simulink model "anfismicrogrid"  (R2017a)
settings: Solver=ode45  StartTime=0.0  StopTime=1  RelTol=1e-3  EnableMultiTasking=on
undefined symbols (not defined in the file or in its folder): idq, idq1, PV1
libraries: powerlib x57, powerlib_meascontrol x5, fuzblock x4, powerlib_extras x3, simulink x1, re_lib x1
(part 1 of 2)
settings Model: Creator=Indhu  LastModifiedBy=venka
settings DataIOCC: LimitDataPoints=on  SaveFormat=Array
settings OptimizationCC: LifeSpan=inf
settings DebuggingCC: SolverPrmCheckMsg=warning  SFUnexpectedBacktrackingDiag=warning  SFNoUnconditionalDefaultTransitionDiag=warning  SFExecutionAtInitializationDiag=none
settings HardwareCC: ProdBitPerPointer=32  ProdBitPerSizeT=32  ProdBitPerPtrDiffT=32  ProdLargestAtomicFloat=None  ProdIntDivRoundTo=Undefined  ProdEndianess=Unspecified  ProdWordSize=32  ProdHWDeviceType=32-bit Generic
settings ModelReferenceCC: PropagateSignalLabelsOutOfModel=off
settings GRTTargetCC: TargetLangStandard=C89/C90 (ANSI)  GeneratePreprocessorConditionals=Disable all
settings ConfigComp: CovMetricSettings=dw  CovHtmlReporting=on  CovSaveCumulativeToWorkspaceVar=on  CovSaveSingleToWorkspaceVar=on  CovExternalEMLEnable=off  CovSFcnEnable=off

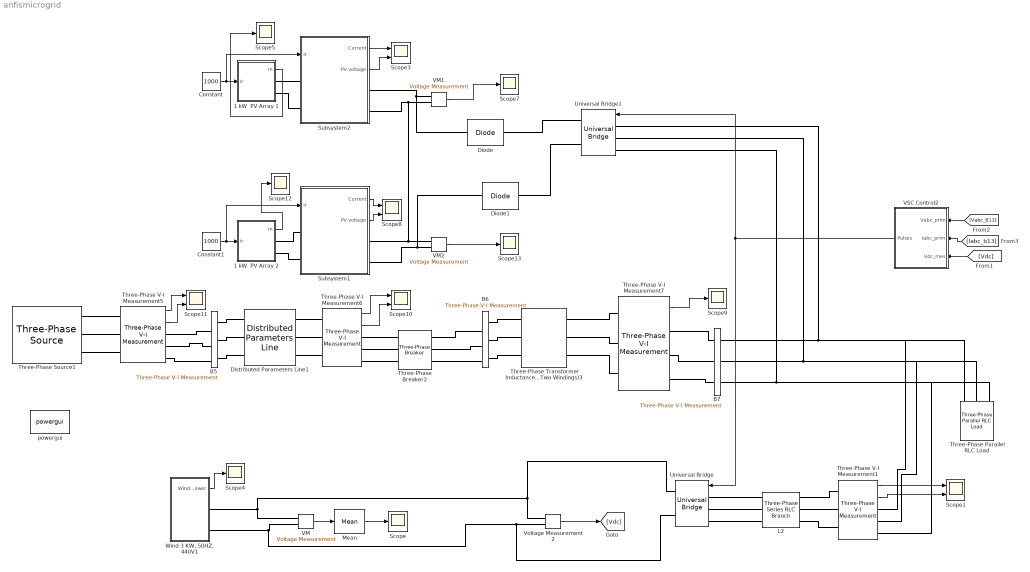
== system anfismicrogrid ==
  1 kW  PV Array 1 : Subsystem  mask(PV array){ModuleType=Suntech STP270S-24_Vb, Ncell=72, Nser=2, Npar=50, ModuleParameters=[ 44.4999  8.19978  35  7.70979 ], ModelParameters=[ 0.32025  2562.3  8.8992e-07  8.2979  1.5 ], Ts=10, PlotVI_module=off, PlotVI_array=off}
      mask prompts: ModuleType "Module type:"; Ncell "Number of cells per module"; Nser "Number of series-connected  modules per string"; Npar "Number of parallel strings"; ModuleParameters "Module specifications under STC  [  Voc, Isc, Vmp, Imp ]"; ModelParameters "Model parameters for 1 module [ Rs, Rp, Isat, Iph, Qd ]"; Ts "Sample time"; PlotVI_module "Display  I-V and  P-V characteritics of one module"; PlotVI_array "Display  I-V and  P-V characteritics of array"
      mask help:
      | Model a PV array
      |
      | PV array consists of Npar strings of modules connected in parallel, each string consisting of Nser modules connected in series.
      |
      | The four PV model parameters (photo-generated current Iph, diode saturation current Isat, parallel resistance Rp and  series resistance Rs) are adjuted to fit the following four module characteristics measured under standard test conditions (STC : irradiance 1000 W/m^2, cell temperature=25 deg. C) and assuming a given "diode quality factor" (Qd) for the semiconductor:
      |   Voc = open circuit voltage
      |   Isc = short-circuit current
      |   Vmp,Imp = voltage and current at maximum power point
      |
      | Select a 'Module type' and then press Apply to see module parameters.
      | Note: Module characteristics are extracted from NREL System Advisor Model.
      mask init:
      | BlockName=gcb;
      | 
      | % SolarModuleSpec_Definition_v2.m
      | %================================
      | %
      | Type=1;
      | SolarModuleSpec(Type).Desc= 'Kyocera KD135GX-LP';
      | SolarModuleSpec(Type).nCells= 36;              % Number of cells in series
      | SolarModuleSpec(Type).Pmp= 135.044;            % Maximum power (W)
      | SolarModuleSpec(Type).Vmp= 17.7;               % Maximum power voltage (V) 
      | SolarModuleSpec(Type).Imp= 7.62959;            % Maximum power current (A)
      | SolarModuleSpec(Type).Voc= 22.0999;            % Open circuit voltage (V)
      | SolarModuleSpec(Type).Isc= 8.36955;            % Short circuit current (A)
      | SolarModuleSpec(Type).TempC_Pmp= -6.445e-001;  % Maximum power temp. coefficient (W/deg.C)
      | SolarModuleSpec(Type).TempC_Vmp= -8.200e-002;  % Maximum power voltage temp. coefficient (V/deg.C)
      | SolarModuleSpec(Type).TempC_Imp= -1.068e-003;  % Maximum power current temp. coefficient (A/deg.C
      | SolarModuleSpec(Type).TempC_Voc= -8.000e-002;  % Open circuit voltage temp. coefficient (V/deg.C)
      | SolarModuleSpec(Type).TempC_Isc= 5.022e-003;   % Short circuit current temp. coefficient (A/deg.C)
      | SolarModuleSpec(Type).Rs= 0.10593;             % Series resistance of PV model (ohms)
      | SolarModuleSpec(Type).Rp= 142.84;              % Parallel resistance of PV model (ohms)
      | SolarModuleSpec(Type).Isat= 9.845e-07;         % Diode saturation current of PV model (A)
      | SolarModuleSpec(Type).Iph=  8.3758;            % Light-generated photo-current  of PV model (A)
      | SolarModuleSpec(Type).Qd= 1.5;                 % Diode quality factor of PV model
      | %-------------------------------------------------------------------------
      | %
      | Type=2;
      | SolarModuleSpec(Type).Desc= 'Kyocera KD205GX-LP';
      | SolarModuleSpec(Type).nCells= 54;              % Number of cells in series
      | SolarModuleSpec(Type).Pmp= 205.075;            % Maximum power (W)
      | SolarModuleSpec(Type).Vmp= 26.6;               % Maximum power voltage (V) 
      | SolarModuleSpec(Type).Imp= 7.70959;            % Maximum power current (A)
      | SolarModuleSpec(Type).Voc= 33.1999;            % Open circuit voltage (V)
      | SolarModuleSpec(Type).Isc= 8.35955;            % Short circuit current (A)
      | SolarModuleSpec(Type).TempC_Pmp= -9.770e-001;  % Maximum power temp. coefficient (W/deg.C)
      | SolarModuleSpec(Type).TempC_Vmp= -1.230e-001;  % Maximum power voltage temp. coefficient (V/deg.C)
      | SolarModuleSpec(Type).TempC_Imp= -1.079e-003;  % Maximum power current temp. coefficient (A/deg.C
      | SolarModuleSpec(Type).TempC_Voc= -1.200e-001;  % Open circuit voltage temp. coefficient (V/deg.C)
      | SolarModuleSpec(Type).TempC_Isc= 5.016e-003;   % Short circuit current temp. coefficient (A/deg.C)
      | SolarModuleSpec(Type).Rs= 0.15945;             % Series resistance of PV model (ohms)
      | SolarModuleSpec(Type).Rp= 1010.6;              % Parallel resistance of PV model (ohms)
      | SolarModuleSpec(Type).Isat=  9.7399e-07;       % Diode saturation current of PV model (A)
      | SolarModuleSpec(Type).Iph= 8.3642;             % Light-generated photo-current  of PV model (A)
      | SolarModuleSpec(Type).Qd= 1.5;                 % Diode quality factor of PV model
      | %-------------------------------------------------------------------------
      | %
      | Type=3;
      | SolarModuleSpec(Type).Desc= 'Mitsubishi PV-UD190MF5';
      | SolarModuleSpec(Type).nCells= 50;              % Number of cells in series
      | SolarModuleSpec(Type).Pmp= 190.503;            % Maximum power (W)
      | SolarModuleSpec(Type).Vmp= 24.6999;            % Maximum power voltage (V) 
      | SolarModuleSpec(Type).Imp= 7.71272;            % Maximum power current (A)
      | SolarModuleSpec(Type).Voc= 30.8006;            % Open circuit voltage (V)
      | SolarModuleSpec(Type).Isc= 8.23289;            % Short circuit current (A)
      | SolarModuleSpec(Type).TempC_Pmp= -8.597e-001;  % Maximum power temp. coefficient (W/deg.C)
      | SolarModuleSpec(Type).TempC_Vmp= -1.090e-001;  % Maximum power voltage temp. coefficient (V/deg.C)
      | SolarModuleSpec(Type).TempC_Imp= -7.713e-004;  % Maximum power current temp. coefficient (A/deg.C
      | SolarModuleSpec(Type).TempC_Voc= -1.050e-001;  % Open circuit voltage temp. coefficient (V/deg.C)
      | SolarModuleSpec(Type).TempC_Isc= 4.446e-003;   % Short circuit current temp. coefficient (A/deg.C)
      | SolarModuleSpec(Type).Rs= 0.20758;             % Series resistance of PV model (ohms)
      | SolarModuleSpec(Type).Rp= 975.6;               % Parallel resistance of PV model (ohms)
      | SolarModuleSpec(Type).Isat= 7.9676e-08;        % Diode saturation current of PV model (A)
      | SolarModuleSpec(Type).Iph= 8.2649;             % Light-generated photo-current  of PV model (A)
      | SolarModuleSpec(Type).Qd= 1.3;                 % Diode quality factor of PV model
      | %-------------------------------------------------------------------------
      | %
      | Type=4;
      | SolarModuleSpec(Type).Desc= 'Sanyo HIP-225HDE1';
      | SolarModuleSpec(Type).nCells= 60;              % Number of cells in series
      | SolarModuleSpec(Type).Pmp= 224.899;            % Maximum power (W)
      | SolarModuleSpec(Type).Vmp= 33.9;               % Maximum power voltage (V) 
      | SolarModuleSpec(Type).Imp= 6.63419;            % Maximum power current (A)
      | SolarModuleSpec(Type).Voc= 41.7984;            % Open circuit voltage (V)
      | SolarModuleSpec(Type).Isc= 7.13383;            % Short circuit current (A)
      | SolarModuleSpec(Type).TempC_Pmp= -6.925e-001;  % Maximum power temp. coefficient (W/deg.C)
      | SolarModuleSpec(Type).TempC_Vmp= -1.010e-001;  % Maximum power voltage temp. coefficient (V/deg.C)
      | SolarModuleSpec(Type).TempC_Imp= -6.634e-004;  % Maximum power current temp. coefficient (A/deg.C
      | SolarModuleSpec(Type).TempC_Voc= -1.050e-001;  % Open circuit voltage temp. coefficient (V/deg.C)
      | SolarModuleSpec(Type).TempC_Isc= 2.140e-003;   % Short circuit current temp. coefficient (A/deg.C)
      | SolarModuleSpec(Type).Rs=  0.20439;            % Series resistance of PV model (ohms)
      | SolarModuleSpec(Type).Rp= 1830.7;              % Parallel resistance of PV model (ohms)
      | SolarModuleSpec(Type).Isat=  3.0815e-07;       % Diode saturation current of PV model (A)
      | SolarModuleSpec(Type).Iph=  7.145;             % Light-generated photo-current  of PV model (A)
      | SolarModuleSpec(Type).Qd= 1.6;                 % Diode quality factor of PV model
      | %-------------------------------------------------------------------------
      | %
      | 
      | Type=5;
      | % NREL : 2007(E)
      | SolarModuleSpec(Type).Desc= 'SunPower SPR-305-WHT';
      | SolarModuleSpec(Type).nCells= 96;              % Number of cells in series
      | SolarModuleSpec(Type).Pmp= 305.2;              % Maximum power (W)
      | SolarModuleSpec(Type).Vmp= 54.70;              % Maximum power voltage (V) 
      | SolarModuleSpec(Type).Imp= 5.58;               % Maximum power current (A)
      | SolarModuleSpec(Type).Voc= 64.20;              % Open circuit voltage (V)
      | SolarModuleSpec(Type).Isc= 5.96;               % Short circuit current (A)
      | SolarModuleSpec(Type).TempC_Pmp= -1.154e+000;  % Maximum power temp. coefficient (W/deg.C)
      | SolarModuleSpec(Type).TempC_Vmp= -1.860e-001;  % Maximum power voltage temp. coefficient (V/deg.C)
      | SolarModuleSpec(Type).TempC_Imp= -2.120e-003;  % Maximum power current temp. coefficient (A/deg.C
      | SolarModuleSpec(Type).TempC_Voc= -1.770e-001;  % Open circuit voltage temp. coefficient (V/deg.C)
      | SolarModuleSpec(Type).TempC_Isc= 3.516e-003;   % Short circuit current temp. coefficient (A/deg.C)
      | SolarModuleSpec(Type).Rs= 0.037998;            % Series resistance of PV model (ohms)
      | SolarModuleSpec(Type).Rp= 993.51;              % Parallel resistance of PV model (ohms)
      | SolarModuleSpec(Type).Isat= 1.1753e-08;        % Diode saturation current of PV model (A)
      | SolarModuleSpec(Type).Iph= 5.9602;             % Light-generated photo-current  of PV model (A)
      | SolarModuleSpec(Type).Qd= 1.3;                 % Diode quality factor of PV model
      | %-------------------------------------------------------------------------
      | %
      | Type=6;
      | SolarModuleSpec(Type).Desc= 'Suntech STP270S-24_Vb';
      | SolarModuleSpec(Type).nCells= 72;              % Number of cells in series
      | SolarModuleSpec(Type).Pmp= 269.843;            % Maximum power (W)
      | SolarModuleSpec(Type).Vmp= 35;                 % Maximum power voltage (V) 
      | SolarModuleSpec(Type).Imp= 7.70979;            % Maximum power current (A)
      | SolarModuleSpec(Type).Voc= 44.4999;            % Open circuit voltage (V)
      | SolarModuleSpec(Type).Isc= 8.19978;            % Short circuit current (A)
      | SolarModuleSpec(Type).TempC_Pmp= -1.204e+000;  % Maximum power temp. coefficient (W/deg.C)
      | SolarModuleSpec(Type).TempC_Vmp= -1.567e-001;  % Maximum power voltage temp. coefficient (V/deg.C)
      | SolarModuleSpec(Type).TempC_Imp= 1.234e-004;   % Maximum power current temp. coefficient (A/deg.C
      | SolarModuleSpec(Type).TempC_Voc= -1.504e-001;  % Open circuit voltage temp. coefficient (V/deg.C)
      | SolarModuleSpec(Type).TempC_Isc= 4.969e-003;   % Short circuit current temp. coefficient (A/deg.C)
      | SolarModuleSpec(Type).Rs= 0.32025;             % Series resistance of PV model (ohms)
      | SolarModuleSpec(Type).Rp= 2562.3;              % Parallel resistance of PV model (ohms)
      | SolarModuleSpec(Type).Isat= 8.8992e-07;        % Diode saturation current of PV model (A)
      | SolarModuleSpec(Type).Iph= 8.2979;             % Light-generated photo-current  of PV model (A)
      | SolarModuleSpec(Type).Qd= 1.5;                 % Diode quality factor of PV model
      | % 
      | %-------------------------------------------------------------------------
      | %
      | Type=7;
      | SolarModuleSpec(Type).Desc= 'Canadian Solar CS5P-220M';
      | SolarModuleSpec(Type).nCells= 96;              % Number of cells in series
      | SolarModuleSpec(Type).Pmp= 219.72;             % Maximum power (W)
      | SolarModuleSpec(Type).Vmp= 48.3159;            % Maximum power voltage (V) 
      | SolarModuleSpec(Type).Imp= 4.54758;            % Maximum power current (A)
      | SolarModuleSpec(Type).Voc= 59.2618;            % Open circuit voltage (V)
      | SolarModuleSpec(Type).Isc= 5.09261;            % Short circuit current (A)
      | SolarModuleSpec(Type).TempC_Pmp= -1.031e+000;  % Maximum power temp. coefficient (W/deg.C)
      | SolarModuleSpec(Type).TempC_Vmp= -2.355e-001;  % Maximum power voltage temp. coefficient (V/deg.C)
      | SolarModuleSpec(Type).TempC_Imp= 8.231e-004;   % Maximum power current temp. coefficient (A/deg.C
      | SolarModuleSpec(Type).TempC_Voc= -2.170e-001;  % Open circuit voltage temp. coefficient (V/deg.C)
      | SolarModuleSpec(Type).TempC_Isc= 2.022e-003;   % Short circuit current temp. coefficient (A/deg.C)
      | SolarModuleSpec(Type).Rs= 0.24807;             % Series resistance of PV model (ohms)
      | SolarModuleSpec(Type).Rp= 235.76;              % Parallel resistance of PV model (ohms)
      | SolarModuleSpec(Type).Isat= 5.3103e-07;        % Diode saturation current of PV model (A)
      | SolarModuleSpec(Type).Iph= 5.098;              % Light-generated photo-current  of PV model (A)
      | SolarModuleSpec(Type).Qd= 1.5;                 % Diode quality factor of PV model
      | %-------------------------------------------------------------------------
      | %
      | Type=8;
      | SolarModuleSpec(Type).Desc= 'BP Solar SX3190';
      | SolarModuleSpec(Type).nCells= 50;              % Number of cells in series
      | SolarModuleSpec(Type).Pmp= 190.258;            % Maximum power (W)
      | SolarModuleSpec(Type).Vmp= 24.3003;            % Maximum power voltage (V) 
      | SolarModuleSpec(Type).Imp= 7.82945;            % Maximum power current (A)
      | SolarModuleSpec(Type).Voc= 30.6021;            % Open circuit voltage (V)
      | SolarModuleSpec(Type).Isc= 8.51029;            % Short circuit current (A)
      | SolarModuleSpec(Type).TempC_Pmp= -9.306e-001;  % Maximum power temp. coefficient (W/deg.C)
      | SolarModuleSpec(Type).TempC_Vmp= -1.140e-001;  % Maximum power voltage temp. coefficient (V/deg.C)
      | SolarModuleSpec(Type).TempC_Imp= -1.566e-003;  % Maximum power current temp. coefficient (A/deg.C
      | SolarModuleSpec(Type).TempC_Voc= -1.110e-001;  % Open circuit voltage temp. coefficient (V/deg.C)
      | SolarModuleSpec(Type).TempC_Isc= 5.532e-003;   % Short circuit current temp. coefficient (A/deg.C)
      | SolarModuleSpec(Type).Rs= 0.17514;             % Series resistance of PV model (ohms)
      | SolarModuleSpec(Type).Rp= 755.51;              % Parallel resistance of PV model (ohms)
      | SolarModuleSpec(Type).Isat= 1.0647e-06;       % Diode saturation current of PV model (A)
      | SolarModuleSpec(Type).Iph= 8.5158;             % Light-generated photo-current  of PV model (A)
      | SolarModuleSpec(Type).Qd= 1.5;                 % Diode quality factor of PV model
      | %-------------------------------------------------------------------------
      | %
      | Type=9;
      | SolarModuleSpec(Type).Desc= 'First Solar FS-272';
      | SolarModuleSpec(Type).nCells= 116;             % Number of cells in series
      | SolarModuleSpec(Type).Pmp= 71.326;             % Maximum power (W)
      | SolarModuleSpec(Type).Vmp= 70.558;             % Maximum power voltage (V) 
      | SolarModuleSpec(Type).Imp= 1.01088;            % Maximum power current (A)
      | SolarModuleSpec(Type).Voc= 94.5738;            % Open circuit voltage (V)
      | SolarModuleSpec(Type).Isc= 1.18103;            % Short circuit current (A)
      | SolarModuleSpec(Type).TempC_Pmp= -2.332e-001;  % Maximum power temp. coefficient (W/deg.C)
      | SolarModuleSpec(Type).TempC_Vmp= -2.060e-001;  % Maximum power voltage temp. coefficient (V/deg.C)
      | SolarModuleSpec(Type).TempC_Imp= -3.538e-004;  % Maximum power current temp. coefficient (A/deg.C
      | SolarModuleSpec(Type).TempC_Voc= -2.690e-001;  % Open circuit voltage temp. coefficient (V/deg.C)
      | SolarModuleSpec(Type).TempC_Isc= 5.433e-004;   % Short circuit current temp. coefficient (A/deg.C)
      | SolarModuleSpec(Type).Rs= 7.7692;              % Series resistance of PV model (ohms)
      | SolarModuleSpec(Type).Rp= 1044.9;              % Parallel resistance of PV model (ohms)
      | SolarModuleSpec(Type).Isat= 1.1116e-068;       % Diode saturation current of PV model (A)
      | SolarModuleSpec(Type).Iph= 1.1898;             % Light-generated photo-current  of PV model (A)
      | SolarModuleSpec(Type).Qd= 2.3;                 % Diode quality factor of PV model
      | %-------------------------------------------------------------------------
      | %
      | Type=10;
      | SolarModuleSpec(Type).Desc= 'SunPower 128-cell Module';
      | SolarModuleSpec(Type).nCells= 128;             % Number of cells in series
      | SolarModuleSpec(Type).Pmp= 400.048;            % Maximum power (W)
      | SolarModuleSpec(Type).Vmp= 72.8992;            % Maximum power voltage (V) 
      | SolarModuleSpec(Type).Imp= 5.48769;            % Maximum power current (A)
      | SolarModuleSpec(Type).Voc= 85.2983;            % Open circuit voltage (V)
      | SolarModuleSpec(Type).Isc= 5.8675;             % Short circuit current (A)
      | SolarModuleSpec(Type).TempC_Pmp= -1.638e+000;  % Maximum power temp. coefficient (W/deg.C)
      | SolarModuleSpec(Type).TempC_Vmp= -2.760e-001;  % Maximum power voltage temp. coefficient (V/deg.C)
      | SolarModuleSpec(Type).TempC_Imp= -1.690e-003;  % Maximum power current temp. coefficient (A/deg.C
      | SolarModuleSpec(Type).TempC_Voc= -2.664e-001;  % Open circuit voltage temp. coefficient (V/deg.C)
      | SolarModuleSpec(Type).TempC_Isc= 1.837e-003;   % Short circuit current temp. coefficient (A/deg.C)
      | SolarModuleSpec(Type).Rs= 0.12264;             % Series resistance of PV model (ohms)
      | SolarModuleSpec(Type).Rp= 859.93;              % Parallel resistance of PV model (ohms)
      | SolarModuleSpec(Type).Isat= 2.3385e-09;        % Diode saturation current of PV model (A)
      | SolarModuleSpec(Type).Iph= 5.8683;             % Light-generated photo-current  of PV model (A)
      | SolarModuleSpec(Type).Qd= 1.2;                 % Diode quality factor of PV model
      | %-------------------------------------------------------------------------
      | 
      | Type=strmatch(ModuleType,char(SolarModuleSpec.Desc));
      | 
      | k= 1.3806e-23; % Boltzman constant (J.K^-1)
      | q=1.6022e-19;  % electron charge  (C)
      | T=273+25;
      | 
      | nCells=SolarModuleSpec(Type).nCells;
      | Voc=SolarModuleSpec(Type).Voc;
      | Isc=SolarModuleSpec(Type).Isc;
      | Vm=SolarModuleSpec(Type).Vmp;
      | Im=SolarModuleSpec(Type).Imp;
      | 
      | set_param(BlockName,'Ncell',num2str(nCells));
      | str=sprintf('[ %g  %g  %g  %g ]',Voc,Isc,Vm,Im);
      | set_param(BlockName,'ModuleParameters',str);
      | 
      | Rs=SolarModuleSpec(Type).Rs;
      | Rp=SolarModuleSpec(Type).Rp; 
      | Isat=SolarModuleSpec(Type).Isat;
      | Iph=SolarModuleSpec(Type).Iph;            
      | Qd=SolarModuleSpec(Type).Qd;
      | 
      | VT=k*T/q*nCells*Qd;
      | 
      | str=sprintf('[ %g  %g  %g  %g  %g ]',Rs,Rp,Isat,Iph, Qd);
      | set_param(BlockName,'ModelParameters',str)
      | 
      | Iph_array=Iph*Npar;
      | Isat_array=Isat*Npar;
      | VT_array=VT*Nser;
      | Rs_array=Rs*Nser/Npar;
      | Rp_array=Rp*Nser/Npar;
      | %
      | %% Plot I-V & P-V characteristics of one module
      | %==============================================
      | if PlotVI_module | PlotVI_array
      |     assignin('base','Voc',Voc);
      |     assignin('base','Isc',Isc);
      |     assignin('base','Rs',Rs);
      |     assignin('base','Rp',Rp);
      |     assignin('base','Isat',Isat);
      |     assignin('base','VT',VT);
      |      
      |     if PlotVI_module, 
      |         F1=figure('Name','I-V and P-V characteristics of one module at 25 deg.C');
      |     end
      |     if PlotVI_array ,
      |         F2=figure('Name','I-V and P-V characteristics of array at 25 deg.C');  
      |     end
      |     load_system('PV_model_Param');
      |     
      |     for ksun=1:-0.25:0.25
      |         assignin('base','Iph',Iph*ksun)
      |         sim('PV_model_Param');
      |         n=find(I_PV>=0);
      |         I_PV=I_PV(n);
      |         V_PV=V_PV(n);
      |         P_PV=V_PV.*I_PV;
      |         
      |         if PlotVI_module
      |             figure(F1);
      |             subplot(211)
      |             if ksun==1
      |                 plot(V_PV,I_PV,'b',[0  Vm Voc], [Isc Im 0],'ro')
      |                 text(Voc/15,Isc*1.1,'1 kW/m^2')
      |                 hold on
      |                 grid
      |             else
      |                 plot(V_PV,I_PV,'--m')
      |                 text(Voc/15, Isc*(ksun+0.1) , sprintf('%g kW/m^2',ksun))
      |             end
      | 
      |             subplot(212) 
      |             if ksun==1
      |                 plot(V_PV,P_PV,'b',[0  Vm Voc], [0 Im*Vm 0],'ro')
      |                 text(Vm*1.02,Vm*Im,'1 kW/m^2')
      |                 hold on
      |                 grid
      |             else
      |                 n= find(P_PV==max(P_PV));
      |                 plot(V_PV,P_PV,'--m', V_PV(n) , P_PV(n),'mo')
      |                 text(Vm*1.02, Vm*Im*ksun, sprintf('%g kW/m^2',ksun))
      |             end
      |             subplot(211)
      |             ylabel('Current (A)')
      |             xlabel('Voltage (V)')
      |             title(sprintf('Module type: %s',SolarModuleSpec(Type).Desc))
      |             axis_xy=axis;
      |             axis_xy(4)=Isc*1.2;
      |             axis(axis_xy);
      |             
      |             subplot(212)
      |             ylabel('Power (W)')
      |             xlabel('Voltage (V)')
      |             axis_xy=axis;
      |             axis_xy(4)=Vm*Im*1.2;
      |             axis(axis_xy);
      |                   
      |             set_param(BlockName,'PlotVI_module', 'off')
      |         end
      |         
      |         if PlotVI_array
      |             figure(F2);
      |             subplot(211)
      |             if ksun==1
      |                 plot(V_PV*Nser,I_PV*Npar,'b',[0  Vm Voc]*Nser, [Isc Im 0]*Npar,'ro')
      |                 text(Voc/15*Nser,Isc*1.1*Npar,'1 kW/m^2')
      |                 hold on
      |                 grid
      |             else
      |                 plot(V_PV*Nser,I_PV*Npar,'--m')
      |                 text(Voc*Nser/15, Isc*Npar*(ksun+0.1) , sprintf('%g kW/m^2',ksun))
      |             end
      |            
      | 
      |             subplot(212)
      |             if ksun==1
      |                 plot(V_PV*Nser,P_PV*Nser*Npar,'b',[0  Vm Voc]*Nser, [0 Im*Vm 0]*Nser*Npar,'ro')
      |                 text(Vm*Nser*1.02,Vm*Im*Nser*Npar,'1 kW/m^2')
      |                 hold on
      |                 grid
      |             else
      |                 n= find(P_PV==max(P_PV));
      |                 plot(V_PV*Nser,P_PV*Nser*Npar,'--m', V_PV(n)*Nser , P_PV(n)*Nser*Npar,'mo')
      |                 text(Vm*Nser*1.02, Vm*Im*Nser*Npar*ksun, sprintf('%g kW/m^2',ksun))
      |             end 
      |             subplot(211)
      |             ylabel('Current (A)')
      |             xlabel('Voltage (V)')
      |             title(sprintf('Array type: %s; %d series modules; %d parallel strings',SolarModuleSpec(Type).Desc,Nser,Npar));
      |             axis_xy=axis;
      |             axis_xy(4)=Isc*Npar*1.2;
      |             axis(axis_xy);
      |             
      |             subplot(212)
      |             ylabel('Power (W)')
      |             xlabel('Voltage (V)')
      |             xis_xy=axis;
      |             axis_xy(4)=Vm*Im*Nser*Npar*1.2;
      |             axis(axis_xy);
      |             
      |             set_param(BlockName,'PlotVI_array', 'off')
      |         end
      |         
      |     end  
      | end
      mask TypeOptions ModuleType: BP Solar SX3190 | Canadian Solar CS5P-220M | First Solar FS-272 | Kyocera KD135GX-LP | Kyocera KD205GX-LP | Mitsubishi PV-UD190MF5 | Sanyo HIP-225HDE1 | SunPower SPR-305-WHT | SunPower SPR-400-WHT | Suntech STP270S-24_Vb
      mask Display: image(imread('panel.jpg'))
  1 kW  PV Array 2 : Subsystem  mask(PV array){ModuleType=Suntech STP270S-24_Vb, Ncell=72, Nser=2, Npar=50, ModuleParameters=[ 44.4999  8.19978  35  7.70979 ], ModelParameters=[ 0.32025  2562.3  8.8992e-07  8.2979  1.5 ], Ts=10, PlotVI_module=off, PlotVI_array=off}
      mask prompts: ModuleType "Module type:"; Ncell "Number of cells per module"; Nser "Number of series-connected  modules per string"; Npar "Number of parallel strings"; ModuleParameters "Module specifications under STC  [  Voc, Isc, Vmp, Imp ]"; ModelParameters "Model parameters for 1 module [ Rs, Rp, Isat, Iph, Qd ]"; Ts "Sample time"; PlotVI_module "Display  I-V and  P-V characteritics of one module"; PlotVI_array "Display  I-V and  P-V characteritics of array"
      mask help:
      | Model a PV array
      |
      | PV array consists of Npar strings of modules connected in parallel, each string consisting of Nser modules connected in series.
      |
      | The four PV model parameters (photo-generated current Iph, diode saturation current Isat, parallel resistance Rp and  series resistance Rs) are adjuted to fit the following four module characteristics measured under standard test conditions (STC : irradiance 1000 W/m^2, cell temperature=25 deg. C) and assuming a given "diode quality factor" (Qd) for the semiconductor:
      |   Voc = open circuit voltage
      |   Isc = short-circuit current
      |   Vmp,Imp = voltage and current at maximum power point
      |
      | Select a 'Module type' and then press Apply to see module parameters.
      | Note: Module characteristics are extracted from NREL System Advisor Model.
      mask init: same as anfismicrogrid/1 kW  PV Array 1
      mask TypeOptions ModuleType: BP Solar SX3190 | Canadian Solar CS5P-220M | First Solar FS-272 | Kyocera KD135GX-LP | Kyocera KD205GX-LP | Mitsubishi PV-UD190MF5 | Sanyo HIP-225HDE1 | SunPower SPR-305-WHT | SunPower SPR-400-WHT | Suntech STP270S-24_Vb
      mask Display: image(imread('panel.jpg'))
  B5 : powerlib/Measurements/Three-Phase V-I Measurement  VoltageMeasurement=phase-to-ground  SetLabelV=off  LabelV=Vabc_B12  Vpu=off  VpuLL=off  CurrentMeasurement=no  SetLabelI=off  LabelI=A1  Ipu=off  Pbase=100e6  Vbase=25e3  OutputType=Magnitude  PhasorSimulation=off  PSBequivalent=0
  B6 : powerlib/Measurements/Three-Phase V-I Measurement  VoltageMeasurement=phase-to-phase  SetLabelV=off  LabelV=Vabc_B12  Vpu=off  VpuLL=off  CurrentMeasurement=no  SetLabelI=off  LabelI=A1  Ipu=off  Pbase=100e6  Vbase=440  OutputType=Magnitude  PhasorSimulation=off  PSBequivalent=0
  B7 : powerlib/Measurements/Three-Phase V-I Measurement  VoltageMeasurement=phase-to-ground  SetLabelV=on  LabelV=Vabc_B13  Vpu=off  VpuLL=off  CurrentMeasurement=yes  SetLabelI=on  LabelI=Iabc_b13  Ipu=off  Pbase=100e6  Vbase=440  OutputType=Magnitude  PhasorSimulation=off  PSBequivalent=0
  Constant : Constant  Value=1000
  Constant1 : Constant  Value=1000
  Diode : powerlib/Power Electronics/Diode  Ron=0.001  Lon=0  Vf=0.8  IC=0  UseSnubber=off  Rs=500  Cs=250e-9  Measurements=off
  Diode1 : powerlib/Power Electronics/Diode  Ron=0.001  Lon=0  Vf=0.8  IC=0  UseSnubber=off  Rs=500  Cs=250e-9  Measurements=off
  Distributed Parameters Line1 : powerlib/Elements/Distributed Parameters Line  Phases=3  Frequency=50  Resistance=[0.01273 0.3864]  Inductance="[0.9337e-3  4.1264e-3]"  Capacitance=[12.74e-9 7.751e-9]  Length=100  x1=[-0.000566 1.22888331647929e-09 21692.7856056922 -60791.8490491303;-0.000565 1.22816301093646e-09 21711.8828575191 -60785.0310596955;-0.000564 1.22744258417879e-09 21730.9779664691 -60778.2070710186;-0.000563 1.2267220362774e-09 21750.0709306575 -60771.3770837731;-0.000562 1.22600136730339e-09 21769.1617482 -60764.5410986332;-0.000561 1.22528057732791e-09 21788.2504172123 -60757.6991162735;-0.00056 1.22455966642207e-09 21807.3369358105 -60750.8511373693;-0.000559 1.22383863465705e-09 21826.4213021109 -60743.9971625965;-0.000558 1.22311748210399e-09 21845.5035142299 -60737.1371926315;-0.000557 1.22239620883408e-09 21864.5835702841 -60730.2712281514;-0.000556 1.22167481491849e-09 21883.6614683904 -60723.3992698339;-0.000555 1.22095330042844e-09 21902.7372066659 -60716.5213183571;-0.000554 1.22023166543513e-09 21921.8107832279 -60709.6373743999;-0.000553 1.21950991000978e-09 21940.8821961939 -60702.7474386417;-0.000552 1.21878803422363e-09 21959.9514436817 -60695.8515117625;-0.000551 1.21806603814792e-09 21979.0185238092 -60688.9495944429;-0.00055 1.21734392185391e-09 21998.0834346945 -60682.0416873641;-0.000549 1.21662168541288e-09 22017.146174456 -60675.127791208;-0.000548 1.21589932889609e-09 22036.2067412123 -60668.2079066567;-0.000547 1.21517685237486e-09 22055.2651330821 -60661.2820343935;-0.000546 1.21445425592048e-09 22074.3213481846 -60654.3501751017;-0.000545 1.21373153960427e-09 22093.3753846389 -60647.4123294655;-0.000544 1.21300870349756e-09 22112.4272405645 -60640.4684981698;-0.000543 1.21228574767169e-09 22131.476914081 -60633.5186818997;-0.000542 1.21156267219801e-09 22150.5244033083 -60626.5628813412;-0.000541 1.21083947714789e-09 22169.5697063665 -60619.6010971809;-0.00054 1.2101161625927e-09 22188.6128213759 -60612.6333301058;-0.000539 1.20939272860384e-09 22207.653746457 -60605.6595808036;-0.000538 1.2086691752527e-09 22226.6924797305 -60598.6798499627;-0.000537 1.2079455026107e-09 22245.7290193174 -60591.6941382718;-0.000536 1.20722171074925e-09 22264.7633633389 -60584.7024464204;-0.000535 1.2064977997398e-09 22283.7955099164 -60577.7047750986;-0.000534 1.20577376965379e-09 22302.8254571714 -60570.7011249971;-0.000533 1.20504962056268e-09 22321.8532032258 -60563.691496807;-0.000532 1.20432535253794e-09 22340.8787462016 -60556.6758912203;-0.000531 1.20360096565105e-09 22359.9020842211 -60549.6543089292;-0.00053 1.20287645997351e-09 22378.9232154067 -60542.6267506268;-0.000529 1.20215183557683e-09 22397.9421378811 -60535.5932170067;-0.000528 1.20142709253251e-09 22416.9588497672 -60528.5537087631;-0.000527 1.20070223091209e-09 22435.9733491883 -60521.5082265908;-0.000526 1.19997725078712e-09 22454.9856342675 -60514.456771185;-0.000525 1.19925215222914e-09 22473.9957031285 -60507.3993432418;-0.000524 1.19852693530971e-09 22493.003553895 -60500.3359434577;-0.000523 1.19780160010042e-09 22512.0091846911 -60493.2665725299;-0.000522 1.19707614667285e-09 22531.012593641 -60486.191231156;-0.000521 1.1963505750986e-09 22550.0137788691 -60479.1099200343;-0.00052 1.19562488544929e-09 22569.0127385 -60472.0226398638;-0.000519 1.19489907779653e-09 22588.0094706587 -60464.929391344;-0.000518 1.19417315221195e-09 22607.0039734702 -60457.8301751749;-0.000517 1.19344710876721e-09 22625.9962450599 -60450.7249920571;-0.000516 1.19272094753397e-09 22644.9862835533 -60443.613842692;-0.000515 1.19199466858389e-09 22663.9740870761 -60436.4967277813;-0.000514 1.19126827198865e-09 22682.9596537544 -60429.3736480276;-0.000513 1.19054175781994e-09 22701.9429817143 -60422.2446041338;-0.000512 1.18981512614947e-09 22720.9240690823 -60415.1095968035;-0.000511 1.18908837704896e-09 22739.9029139849 -60407.968626741;-0.00051 1.18836151059013e-09 22758.8795145491 -60400.821694651;-0.000509 1.18763452684472e-09 22777.853868902 -60393.6688012388;-0.000508 1.18690742588449e-09 22796.8259751708 -60386.5099472106;-0.000507 1.18618020778118e-09 22815.7958314831 -60379.3451332727;-0.000506 1.18545287260659e-09 22834.7634359666 -60372.1743601324 ...(+33000 chars)]  x2=[-0.000566 6.32336565604892e-09 21774.1662944161 -61162.7815963556;-0.000565 6.32048140196208e-09 21793.3800741217 -61155.938022119;-0.000564 6.31759652406873e-09 21812.5917029068 -61149.0884120333;-0.000563 6.31471102265361e-09 21831.8011788755 -61142.2327667745;-0.000562 6.31182489800149e-09 21851.0085001317 -61135.3710870193;-0.000561 6.30893815039723e-09 21870.2136647799 -61128.5033734448;-0.00056 6.30605078012574e-09 21889.4166709245 -61121.629626729;-0.000559 6.30316278747198e-09 21908.6175166703 -61114.7498475501;-0.000558 6.300274172721e-09 21927.8162001223 -61107.8640365873;-0.000557 6.29738493615789e-09 21947.0127193856 -61100.9721945201;-0.000556 6.2944950780678e-09 21966.2070725655 -61094.0743220286;-0.000555 6.29160459873596e-09 21985.3992577677 -61087.1704197938;-0.000554 6.28871349844763e-09 22004.589273098 -61080.260488497;-0.000553 6.28582177748817e-09 22023.7771166625 -61073.3445288201;-0.000552 6.28292943614296e-09 22042.9627865672 -61066.4225414458;-0.000551 6.28003647469749e-09 22062.1462809188 -61059.4945270572;-0.00055 6.27714289343726e-09 22081.3275978238 -61052.5604863381;-0.000549 6.27424869264787e-09 22100.5067353891 -61045.6204199729;-0.000548 6.27135387261495e-09 22119.6836917219 -61038.6743286464;-0.000547 6.26845843362422e-09 22138.8584649294 -61031.7222130443;-0.000546 6.26556237596145e-09 22158.0310531192 -61024.7640738528;-0.000545 6.26266569991247e-09 22177.201454399 -61017.7999117585;-0.000544 6.25976840576315e-09 22196.3696668767 -61010.8297274487;-0.000543 6.25687049379947e-09 22215.5356886607 -61003.8535216115;-0.000542 6.25397196430743e-09 22234.6995178591 -60996.8712949353;-0.000541 6.25107281757309e-09 22253.8611525807 -60989.8830481093;-0.00054 6.24817305388261e-09 22273.0205909342 -60982.8887818231;-0.000539 6.24527267352217e-09 22292.1778310287 -60975.8884967671;-0.000538 6.24237167677802e-09 22311.3328709735 -60968.8821936322;-0.000537 6.2394700639365e-09 22330.485708878 -60961.8698731099;-0.000536 6.23656783528396e-09 22349.6363428519 -60954.8515358922;-0.000535 6.23366499110686e-09 22368.7847710052 -60947.8271826719;-0.000534 6.23076153169168e-09 22387.9309914479 -60940.7968141421;-0.000533 6.227857457325e-09 22407.0750022904 -60933.7604309969;-0.000532 6.22495276829343e-09 22426.2168016432 -60926.7180339306;-0.000531 6.22204746488365e-09 22445.3563876172 -60919.6696236383;-0.00053 6.21914154738241e-09 22464.4937583234 -60912.6152008157;-0.000529 6.2162350160765e-09 22483.6289118728 -60905.5547661589;-0.000528 6.2133278712528e-09 22502.7618463771 -60898.4883203649;-0.000527 6.21042011319821e-09 22521.8925599478 -60891.4158641311;-0.000526 6.20751174219974e-09 22541.0210506969 -60884.3373981555;-0.000525 6.20460275854442e-09 22560.1473167363 -60877.2529231366;-0.000524 6.20169316251935e-09 22579.2713561785 -60870.1624397738;-0.000523 6.19878295441172e-09 22598.3931671359 -60863.0659487668;-0.000522 6.19587213450873e-09 22617.5127477214 -60855.963450816;-0.000521 6.19296070309767e-09 22636.6300960478 -60848.8549466224;-0.00052 6.1900486604659e-09 22655.7452102284 -60841.7404368876;-0.000519 6.18713600690082e-09 22674.8580883766 -60834.6199223138;-0.000518 6.1842227426899e-09 22693.9687286061 -60827.4934036036;-0.000517 6.18130886812066e-09 22713.0771290306 -60820.3608814606;-0.000516 6.1783943834807e-09 22732.1832877642 -60813.2223565886;-0.000515 6.17547928905765e-09 22751.2872029214 -60806.0778296922;-0.000514 6.17256358513924e-09 22770.3888726165 -60798.9273014765;-0.000513 6.16964727201322e-09 22789.4882949643 -60791.7707726472;-0.000512 6.16673034996743e-09 22808.5854680798 -60784.6082439107;-0.000511 6.16381281928975e-09 22827.6803900781 -60777.4397159739;-0.00051 6.16089468026814e-09 22846.7730590748 -60770.2651895442;-0.000509 6.1579759331906e-09 22865.8634731853 -60763.0846653299;-0.000508 6.1550565783452e-09 22884.9516305256 -60755.8981440395;-0.000507 6.15213661602008e-09 22904.0375292117 -60748.7056263824;-0.000506 6.14921604650341e-09 22923.1211673599 ...(+33027 chars)]  x3=[-0.000566 6.01701614172706e-11 55.2019150655102 -231.415196710785;-0.000565 6.01759172269448e-11 55.2746135684006 -231.397843098105;-0.000564 6.0181667097494e-11 55.3473066159054 -231.380466647373;-0.000563 6.01874110283509e-11 55.41999420085 -231.363067360305;-0.000562 6.01931490189484e-11 55.4926763160604 -231.345645238617;-0.000561 6.01988810687203e-11 55.5653529543633 -231.32820028403;-0.00056 6.02046071771008e-11 55.6380241085857 -231.310732498264;-0.000559 6.02103273435249e-11 55.7106897715552 -231.293241883045;-0.000558 6.02160415674278e-11 55.7833499361001 -231.275728440097;-0.000557 6.02217498482457e-11 55.8560045950492 -231.258192171151;-0.000556 6.02274521854152e-11 55.9286537412315 -231.240633077936;-0.000555 6.02331485783735e-11 56.0012973674771 -231.223051162185;-0.000554 6.02388390265583e-11 56.0739354666161 -231.205446425634;-0.000553 6.02445235294081e-11 56.1465680314796 -231.18781887002;-0.000552 6.02502020863618e-11 56.219195054899 -231.170168497084;-0.000551 6.02558746968589e-11 56.2918165297064 -231.152495308566;-0.00055 6.02615413603396e-11 56.3644324487341 -231.134799306212;-0.000549 6.02672020762446e-11 56.4370428048154 -231.117080491768;-0.000548 6.02728568440153e-11 56.5096475907839 -231.099338866982;-0.000547 6.02785056630934e-11 56.5822467994737 -231.081574433606;-0.000546 6.02841485329216e-11 56.6548404237197 -231.063787193393;-0.000545 6.02897854529428e-11 56.7274284563571 -231.045977148098;-0.000544 6.02954164226008e-11 56.8000108902218 -231.02814429948;-0.000543 6.03010414413397e-11 56.8725877181501 -231.010288649298;-0.000542 6.03066605086045e-11 56.9451589329791 -230.992410199315;-0.000541 6.03122736238405e-11 57.0177245275462 -230.974508951294;-0.00054 6.03178807864937e-11 57.0902844946895 -230.956584907004;-0.000539 6.03234819960108e-11 57.1628388272476 -230.938638068212;-0.000538 6.03290772518388e-11 57.2353875180597 -230.920668436691;-0.000537 6.03346665534257e-11 57.3079305599656 -230.902676014213;-0.000536 6.03402499002197e-11 57.3804679458054 -230.884660802555;-0.000535 6.03458272916697e-11 57.4529996684201 -230.866622803495;-0.000534 6.03513987272255e-11 57.5255257206511 -230.848562018812;-0.000533 6.03569642063369e-11 57.5980460953402 -230.830478450289;-0.000532 6.03625237284548e-11 57.6705607853302 -230.812372099712;-0.000531 6.03680772930305e-11 57.743069783464 -230.794242968867;-0.00053 6.03736248995158e-11 57.8155730825852 -230.776091059543;-0.000529 6.03791665473631e-11 57.8880706755382 -230.757916373533;-0.000528 6.03847022360257e-11 57.9605625551677 -230.739718912629;-0.000527 6.03902319649571e-11 58.0330487143189 -230.721498678627;-0.000526 6.03957557336115e-11 58.1055291458379 -230.703255673327;-0.000525 6.04012735414439e-11 58.1780038425711 -230.684989898528;-0.000524 6.04067853879095e-11 58.2504727973655 -230.666701356034;-0.000523 6.04122912724644e-11 58.3229360030687 -230.648390047648;-0.000522 6.04177911945653e-11 58.3953934525289 -230.63005597518;-0.000521 6.04232851536691e-11 58.4678451385948 -230.611699140437;-0.00052 6.04287731492339e-11 58.5402910541157 -230.593319545232;-0.000519 6.04342551807178e-11 58.6127311919416 -230.574917191379;-0.000518 6.04397312475798e-11 58.6851655449228 -230.556492080694;-0.000517 6.04452013492796e-11 58.7575941059104 -230.538044214995;-0.000516 6.04506654852771e-11 58.8300168677559 -230.519573596104;-0.000515 6.04561236550331e-11 58.9024338233115 -230.501080225843;-0.000514 6.0461575858009e-11 58.97484496543 -230.482564106037;-0.000513 6.04670220936665e-11 59.0472502869647 -230.464025238514;-0.000512 6.04724623614682e-11 59.1196497807693 -230.445463625104;-0.000511 6.04778966608772e-11 59.1920434396985 -230.426879267638;-0.00051 6.04833249913571e-11 59.2644312566072 -230.408272167952;-0.000509 6.04887473523721e-11 59.336813224351 -230.38964232788;-0.000508 6.04941637433871e-11 59.4091893357862 -230.370989749262;-0.000507 6.04995741638674e-11 59.4815595837694 -230.352314433939;-0.000506 6.05049786132792e-11 59.553923961158 ...(+32966 chars)]  x4=[-0.000566 -4.8868131193548e-11 80.4214138552796 -226.168240383572;-0.000565 -4.88783025583965e-11 80.4924627337196 -226.142964090736;-0.000564 -4.88884690991499e-11 80.5635036678721 -226.117665478485;-0.000563 -4.88986308148049e-11 80.6345366507254 -226.092344549315;-0.000562 -4.89087877043584e-11 80.7055616752691 -226.067001305725;-0.000561 -4.89189397668082e-11 80.7765787344932 -226.041635750216;-0.00056 -4.89290870011521e-11 80.8475878213885 -226.016247885293;-0.000559 -4.89392294063888e-11 80.9185889289469 -225.99083771346;-0.000558 -4.89493669815172e-11 80.9895820501606 -225.965405237226;-0.000557 -4.89594997255367e-11 81.0605671780232 -225.9399504591;-0.000556 -4.89696276374474e-11 81.1315443055284 -225.914473381595;-0.000555 -4.89797507162495e-11 81.2025134256713 -225.888974007226;-0.000554 -4.89898689609441e-11 81.2734745314474 -225.863452338508;-0.000553 -4.89999823705324e-11 81.3444276158531 -225.837908377962;-0.000552 -4.90100909440164e-11 81.4153726718857 -225.812342128108;-0.000551 -4.90201946803983e-11 81.4863096925432 -225.786753591469;-0.00055 -4.90302935786809e-11 81.5572386708242 -225.76114277057;-0.000549 -4.90403876378676e-11 81.6281595997286 -225.735509667941;-0.000548 -4.90504768569621e-11 81.6990724722566 -225.709854286109;-0.000547 -4.90605612349686e-11 81.7699772814094 -225.684176627608;-0.000546 -4.90706407708918e-11 81.840874020189 -225.658476694972;-0.000545 -4.90807154637369e-11 81.9117626815982 -225.632754490737;-0.000544 -4.90907853125096e-11 81.9826432586405 -225.607010017442;-0.000543 -4.91008503162161e-11 82.0535157443203 -225.581243277628;-0.000542 -4.91109104738629e-11 82.1243801316427 -225.555454273838;-0.000541 -4.91209657844571e-11 82.1952364136138 -225.529643008616;-0.00054 -4.91310162470064e-11 82.2660845832403 -225.503809484512;-0.000539 -4.91410618605188e-11 82.3369246335297 -225.477953704074;-0.000538 -4.91511026240029e-11 82.4077565574905 -225.452075669853;-0.000537 -4.91611385364676e-11 82.4785803481318 -225.426175384405;-0.000536 -4.91711695969224e-11 82.5493959984635 -225.400252850286;-0.000535 -4.91811958043773e-11 82.6202035014965 -225.374308070053;-0.000534 -4.91912171578429e-11 82.6910028502424 -225.348341046268;-0.000533 -4.92012336563299e-11 82.7617940377134 -225.322351781494;-0.000532 -4.92112452988499e-11 82.8325770569228 -225.296340278294;-0.000531 -4.92212520844146e-11 82.9033519008846 -225.270306539238;-0.00053 -4.92312540120366e-11 82.9741185626137 -225.244250566893;-0.000529 -4.92412510807285e-11 83.0448770351255 -225.218172363833;-0.000528 -4.92512432895038e-11 83.1156273114366 -225.192071932629;-0.000527 -4.92612306373763e-11 83.1863693845641 -225.16594927586;-0.000526 -4.92712131233603e-11 83.2571032475261 -225.139804396102;-0.000525 -4.92811907464704e-11 83.3278288933414 -225.113637295936;-0.000524 -4.92911635057221e-11 83.3985463150298 -225.087447977945;-0.000523 -4.93011314001309e-11 83.4692555056116 -225.061236444713;-0.000522 -4.93110944287131e-11 83.5399564581082 -225.035002698828;-0.000521 -4.93210525904855e-11 83.6106491655416 -225.008746742879;-0.00052 -4.93310058844651e-11 83.6813336209348 -224.982468579457;-0.000519 -4.93409543096696e-11 83.7520098173115 -224.956168211155;-0.000518 -4.93508978651171e-11 83.8226777476962 -224.929845640569;-0.000517 -4.93608365498263e-11 83.8933374051143 -224.903500870298;-0.000516 -4.93707703628162e-11 83.9639887825919 -224.877133902941;-0.000515 -4.93806993031065e-11 84.034631873156 -224.850744741101;-0.000514 -4.93906233697171e-11 84.1052666698345 -224.824333387382;-0.000513 -4.94005425616686e-11 84.175893165656 -224.797899844391;-0.000512 -4.94104568779821e-11 84.2465113536498 -224.771444114736;-0.000511 -4.9420366317679e-11 84.3171212268464 -224.74496620103;-0.00051 -4.94302708797812e-11 84.3877227782767 -224.718466105884;-0.000509 -4.94401705633113e-11 84.4583160009726 -224.691943831915;-0.000508 -4.94500653672922e-11 84.528900887967 -224.66539938174;-0.000507 -4.94599552907473e-11 84.5994774322933 ...(+33556 chars)]  x5=0.000565541566995743  V1=[0 0 0 2.339e-09 6.456e+04 6.456e+04;0 0 0 314.2 314.2 314.2;1.571 1.571 1.571 -0.9334 0.4129 -1.158]  V2=[0 0 0 9.955e-09 6.494e+04 6.494e+04;0 0 0 314.2 314.2 314.2;1.571 1.571 1.571 -1.047 0.4126 -1.158]  I1=[0 0 0 5.638e-11 239 239;0 0 0 314.2 314.2 314.2;1.571 1.571 1.571 -2.312 0.3045 -1.266]  I2=[0 0 0 5.238e-11 239.1 239.1;0 0 0 314.2 314.2 314.2;1.571 1.571 1.571 0.5382 0.4125 -1.158]  nHarmo=2  Measurements=None
      settings: SourceProductName=Simscape Power Systems
  L2 : powerlib/Elements/Three-Phase Series RLC Branch  LConnTagsString=A|B|C  RConnTagsString=A|B|C  BranchType=LC  Resistance=500e-6*377/50/2  Inductance=2e-2  Capacitance=550e-6  Measurements=None
  Mean : powerlib_meascontrol/Measurements/Mean  Freq=50  Vinit=0  Ts=0
  Scope{,4..5,7,9,12..13} (7 alike) : Scope
  Scope{1,3,8,10..11} (5 alike) : Scope  NumInputPorts=2
  Subsystem1 : Subsystem
  Subsystem2 : Subsystem
  Three-Phase Parallel RLC Load : powerlib/Elements/Three-Phase Parallel RLC Load  LConnTagsString=A|B|C  Configuration=Y (grounded)  NominalVoltage=220  Vabc=[1e3 1e3 1e3]  Vabcp=[1e3 1e3 1e3]  NominalFrequency=50  UnbalancedPower=off  ActivePower=50e3  InductivePower=1000  CapacitivePower=0  Pabc=[10e3 9e3 11e3]  QLabc=[100 90 110]  QCabc=[100 90 110]  Pabcp=[10e3 9e3 11e3]  QLabcp=[100 90 110]  QCabcp=[100 90 110]  Measurements=None  LoadType=constant Z
  Three-Phase V-I Measurement1 : powerlib/Measurements/Three-Phase V-I Measurement  VoltageMeasurement=phase-to-ground  SetLabelV=off  LabelV=Vabc_b1  Vpu=off  VpuLL=off  CurrentMeasurement=yes  SetLabelI=off  LabelI=Iabc_b1  Ipu=off  Pbase=100e6  Vbase=500e3  OutputType=Complex  PhasorSimulation=off  PSBequivalent=0
  Three-Phase V-I Measurement5 : powerlib/Measurements/Three-Phase V-I Measurement  VoltageMeasurement=phase-to-ground  SetLabelV=off  LabelV=Vabc  Vpu=off  VpuLL=off  CurrentMeasurement=yes  SetLabelI=off  LabelI=Iabc  Ipu=off  Pbase=100e6  Vbase=500e3  OutputType=Complex  PhasorSimulation=off  PSBequivalent=0
  Three-Phase V-I Measurement6 : powerlib/Measurements/Three-Phase V-I Measurement  VoltageMeasurement=phase-to-ground  SetLabelV=off  LabelV=Vabc  Vpu=off  VpuLL=off  CurrentMeasurement=yes  SetLabelI=off  LabelI=Iabc  Ipu=off  Pbase=100e6  Vbase=500e3  OutputType=Complex  PhasorSimulation=off  PSBequivalent=0
  Three-Phase V-I Measurement7 : powerlib/Measurements/Three-Phase V-I Measurement  VoltageMeasurement=phase-to-ground  SetLabelV=off  LabelV=Vabc_b1  Vpu=off  VpuLL=off  CurrentMeasurement=no  SetLabelI=off  LabelI=Iabc_b1  Ipu=off  Pbase=100e6  Vbase=500e3  OutputType=Complex  PhasorSimulation=off  PSBequivalent=0
  Three-Phase Breaker2 : powerlib/Elements/Three-Phase Breaker  InitialState=closed  SwitchA=off  SwitchB=off  SwitchC=off  SwitchTimes="[1/50  20/50]"  External=off  BreakerResistance=0.001  SnubberResistance=1e6  SnubberCapacitance=inf  Measurements=None
  Three-Phase Source1 : powerlib/Electrical Sources/Three-Phase Source  InternalConnection=Yg  VoltagePhases=off  Voltage=63510.4  PhaseAngle=0  Voltage_phases=[25e3 25e3 25e3]/sqrt(3)  PhaseAngles_phases=[0 -120 +120]  Frequency=50  NonIdealSource=on  SpecifyImpedance=on  Resistance=0.8929  Inductance=16.58e-3  ShortCircuitLevel=100e6  BaseVoltage=63510.4  XRratio=7  BusType=swing  Pref=0  Qref=0  Prefabc=[10e3, 10e3, 10e3]  Qrefabc=[0, 0, 0]  Qmin=-inf  Qmax=inf
  Three-Phase Transformer Inductance Matrix Type (Two Windings)3 : powerlib/Elements/Three-Phase Transformer Inductance Matrix Type (Two Windings)  CoreType=Three-limb or five-limb core  Winding1Connection=Yg  Winding2Connection=Yg  AutoTransformer=off  Measurements=None  NominalPower=[100e3 50]  VLLnom=[63510.4 254.03]  WindingResistances=[0.01 0.01]  NoLoadIexcPos=2  NoLoadPlossPos=1000  ShortCircuitReactancePos=0.06  ShortCircuitReactancePosAuto=0.06  NoLoadIexcZero=100  NoLoadPlossZero=1500  ShortCircuitReactanceZero=0.03  ShortCircuitReactanceZeroAuto=0.03
      settings: SourceProductName=Simscape Power Systems  SourceProductBaseCode=PS
  Universal Bridge : powerlib/Power Electronics/Universal Bridge  Arms=3  SnubberResistance=1e5  SnubberCapacitance=inf  Device=IGBT / Diodes  Ron=1e-3  Lon=0  ForwardVoltages="[  0  0  ]"  ForwardVoltage=0  GTOparameters=[ 10e-6 , 20e-6 ]  IGBTparameters=[ 1e-6 , 2e-6 ]  Measurements=None  Measurements_2=None  converterType=Rectifier
  Universal Bridge1 : powerlib/Power Electronics/Universal Bridge  Arms=3  SnubberResistance=1e5  SnubberCapacitance=inf  Device=Thyristors  Ron=1e-3  Lon=0  ForwardVoltages="[  0  0  ]"  ForwardVoltage=0  GTOparameters=[ 10e-6 , 20e-6 ]  IGBTparameters=[ 1e-6 , 2e-6 ]  Measurements=None  Measurements_2=None  converterType=Rectifier
  VM : powerlib/Measurements/Voltage Measurement  PhasorSimulation=off  OutputType=Complex  PSBequivalent=0
  VM1 : powerlib/Measurements/Voltage Measurement  PhasorSimulation=off  OutputType=Complex  PSBequivalent=0
  VM2 : powerlib/Measurements/Voltage Measurement  PhasorSimulation=off  OutputType=Complex  PSBequivalent=0
  VSC Control2 : Subsystem  mask(VSC Main Controller){nom=[ 100e3  50 ], Vnom=[ 25e3 260 ], Vnom_dc=220, RLxfo=[0.002  0.06 ], RLchoke=[2e-3  250e-6  ], K_VDCreg=[7  800], K_Ireg=[0.3 20], Ts=1e-6}
      mask prompts: nom "Nominal power and frequency [ Pnom(VA)  Fnom(Hz) ]:"; Vnom "Nominal primary and secondary voltages (Vrms LL) [ Vnom_prim   Vnom_sec ]:"; Vnom_dc "Nominal DC bus voltage (V):"; RLxfo "Total transformer leakage impedance (pu/Pnom) [ Rxfo  Lxf ]"; RLchoke "Choke impedance [ R(ohm) L(H) ]"; K_VDCreg "VDC regultator gains [ Kp  Ki ]:"; K_Ireg "Current regulator gains [ Kp  Ki ]:"; Ts "Sample time"
      mask init:
      | Pnom=nom(1);
      | Fnom=nom(2);
      | Vnom_prim=Vnom(1);
      | Vnom_sec=Vnom(2);
      | Zbase=Vnom_sec^2/Pnom;
      | Rtot_pu=RLxfo(1) + RLchoke(1)/Zbase;
      | Ltot_pu=RLxfo(2) + RLchoke(2)/(Zbase/(2*pi*Fnom));
      | Kp_VDCreg=K_VDCreg(1);
      | Ki_VDCreg=K_VDCreg(2);
      | Kp_Ireg=K_Ireg(1);
      | Ki_Ireg=K_Ireg(2);
      | Vdc_ref=Vnom_dc;
      | % Used to determine initial value of Boost Control (MPPT)
      | assignin('base','Vdc_ref_Inv',Vdc_ref);
  Voltage Measurement2 : powerlib/Measurements/Voltage Measurement  PhasorSimulation=off  OutputType=Complex  PSBequivalent=0
  "Wind 3 KW, 50HZ, 440V1" : Subsystem
  powergui : powerlib/powergui  Priority=1  SimulationMode=Discrete  SampleTime=1e-6  frequency=60  Iterations=50  frequencyindice=0  Pbase=100e6  ErrMax=1e-4  UnitsV=kV  UnitsW=MW  buscounter=0  FunctionMessages=off  echomessages=off  EnableUseOfTLC=off  CurrentSourceSwitches=off  DisableSnubberDevices=off  DisableRonSwitches=off  DisableVfSwitches=off  DisplayEquations=off  SolverType=Tustin  Interpol=off  ExternalGateDelay=off  methode=off  Ts=0  x0status=blocks  SPID=off  SwTol=0  HookPort=off  RestoreLinks=warning  ResistiveCurrentMeasurement=off  Frange=[0:2:500]  Ylog=off  Xlog=on  ShowGrid=off  save=off  variable=ZData  structure=pvg  ZoomFFT=off  StartTime=0.5  cycles=5  DisplayStyle=1  fundamental=50  FreqAxis=off  MaxFrequency=1000  frequencyindicesteady=1  RmsSteady=1  display=off
  wires:
  Three-Phase V-I Measurement6/1 -> Scope10/1
  Three-Phase V-I Measurement6/2 -> Scope10/2
  Three-Phase V-I Measurement5/1 -> Scope11/1
  Three-Phase V-I Measurement5/2 -> Scope11/2
  Voltage Measurement2/1 -> [Vdc]
  Three-Phase V-I Measurement7/1 -> Scope9/1
  Three-Phase V-I Measurement1/1 -> Scope1/1
  Constant/1 -> Subsystem2/1(Ir), 1 kW  PV Array 1/1(Ir)
  Subsystem2/2("PV voltage ") -> Scope3/2
  VM/1 -> Mean/1
  Mean/1 -> Scope/1
  "Wind 3 KW, 50HZ, 440V1"/1(Wind Power) -> Scope4/1
  1 kW  PV Array 1/1(m) -> Scope5/1
  Subsystem2/1("Current ") -> Scope3/1
  [Vabc_B13] -> VSC Control2/1(Vabc_prim)
  [Iabc_b13] -> VSC Control2/2(Iabc_prim)
  [Vdc] -> VSC Control2/3(Vdc_mes)
  VSC Control2/1(Pulses) -> Universal Bridge1/1, Universal Bridge/1
  VM1/1 -> Scope7/1
  Constant1/1 -> 1 kW  PV Array 2/1(Ir), Subsystem1/1(Ir)
  Subsystem1/2("PV voltage ") -> Scope8/2
  1 kW  PV Array 2/1(m) -> Scope12/1
  Subsystem1/1("Current ") -> Scope8/1
  VM2/1 -> Scope13/1
  Three-Phase V-I Measurement1/2 -> Scope1/2
  connections:
  Three-Phase Breaker2/LConn3 -- B6/RConn3
  Three-Phase V-I Measurement6/LConn1 -- Distributed Parameters Line1/RConn1
  Three-Phase V-I Measurement7/RConn3 -- B7/RConn3
  Three-Phase Transformer Inductance Matrix Type (Two Windings)3/LConn1 -- B6/LConn1
  B5/RConn1 -- Three-Phase V-I Measurement5/RConn1
  Three-Phase Source1/RConn3 -- Three-Phase V-I Measurement5/LConn3
  Three-Phase Breaker2/RConn1 -- Three-Phase V-I Measurement6/RConn1
  Three-Phase Source1/RConn1 -- Three-Phase V-I Measurement5/LConn1
  Three-Phase V-I Measurement6/LConn2 -- Distributed Parameters Line1/RConn2
  Three-Phase Transformer Inductance Matrix Type (Two Windings)3/LConn3 -- B6/LConn3
  Three-Phase Breaker2/LConn1 -- B6/RConn1
  Three-Phase Breaker2/LConn2 -- B6/RConn2
  Three-Phase Breaker2/RConn2 -- Three-Phase V-I Measurement6/RConn2
  Three-Phase V-I Measurement6/LConn3 -- Distributed Parameters Line1/RConn3
  Three-Phase Transformer Inductance Matrix Type (Two Windings)3/LConn2 -- B6/LConn2
  Distributed Parameters Line1/LConn1 -- B5/LConn1
  B5/RConn2 -- Three-Phase V-I Measurement5/RConn2
  Three-Phase V-I Measurement7/LConn2 -- Three-Phase Transformer Inductance Matrix Type (Two Windings)3/RConn2
  Three-Phase V-I Measurement7/LConn3 -- Three-Phase Transformer Inductance Matrix Type (Two Windings)3/RConn3
  Distributed Parameters Line1/LConn2 -- B5/LConn2
  Distributed Parameters Line1/LConn3 -- B5/LConn3
  B5/RConn3 -- Three-Phase V-I Measurement5/RConn3
  Three-Phase V-I Measurement7/RConn2 -- B7/RConn2
  Three-Phase Breaker2/RConn3 -- Three-Phase V-I Measurement6/RConn3
  Three-Phase V-I Measurement7/LConn1 -- Three-Phase Transformer Inductance Matrix Type (Two Windings)3/RConn1
  Three-Phase V-I Measurement7/RConn1 -- B7/RConn1
  Three-Phase Source1/RConn2 -- Three-Phase V-I Measurement5/LConn2
  Universal Bridge1/LConn1 -- Three-Phase V-I Measurement1/RConn1 -- Three-Phase Parallel RLC Load/LConn1 -- B7/LConn1
  Universal Bridge1/LConn3 -- Three-Phase V-I Measurement1/RConn3 -- Three-Phase Parallel RLC Load/LConn3 -- B7/LConn3
  Universal Bridge1/LConn2 -- Three-Phase V-I Measurement1/RConn2 -- Three-Phase Parallel RLC Load/LConn2 -- B7/LConn2
  Universal Bridge/LConn1 -- L2/LConn1
  Universal Bridge/LConn2 -- L2/LConn2
  Universal Bridge/LConn3 -- L2/LConn3
  Voltage Measurement2/LConn1 -- VM/LConn1 -- "Wind 3 KW, 50HZ, 440V1"/RConn1 -- Universal Bridge/RConn1
  Voltage Measurement2/LConn2 -- VM/LConn2 -- "Wind 3 KW, 50HZ, 440V1"/RConn2 -- Universal Bridge/RConn2
  Subsystem1/RConn1 -- VM2/LConn1 -- Subsystem2/RConn2 -- VM1/LConn2
  1 kW  PV Array 1/RConn2 -- Subsystem2/LConn2
  1 kW  PV Array 1/RConn1 -- Subsystem2/LConn1
  Subsystem2/RConn1 -- Diode/LConn1 -- VM1/LConn1
  1 kW  PV Array 2/RConn1 -- Subsystem1/LConn1
  Subsystem1/RConn2 -- Diode1/LConn1 -- VM2/LConn2
  1 kW  PV Array 2/RConn2 -- Subsystem1/LConn2
  Diode/RConn1 -- Universal Bridge1/RConn1
  Diode1/RConn1 -- Universal Bridge1/RConn2
  Three-Phase V-I Measurement1/LConn2 -- L2/RConn2
  L2/RConn1 -- Three-Phase V-I Measurement1/LConn1
  L2/RConn3 -- Three-Phase V-I Measurement1/LConn3
